simulink model "motor_cc_velocidade_teste"  (R2017b)
settings: Solver=VariableStepAuto  StartTime=0.0  StopTime=10.0  RelTol=1e-3
values from neighbouring files (symbols this model uses):
  b = 0.1    [motor.m]
  J = 0.01    [motor.m]
  Ke = 0.01    [motor.m]
  Kt = 0.01    [motor.m]
  L = 0.5    [motor.m]
  R = 1    [motor.m]
settings Model: Creator=fernandopassold  LastModifiedBy=fernandopassold

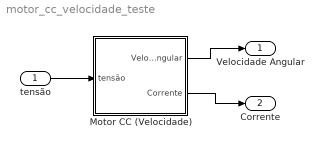
== system motor_cc_velocidade_teste ==
  tensão : Inport
  Motor CC (Velocidade) : Subsystem
  Velocidade Angular : Outport
  Corrente : Outport  Port=2
  wires:
  tensão/1 -> Motor CC (Velocidade)/1(tensão)
  Motor CC (Velocidade)/1(Velocidade Angular) -> Velocidade Angular/1
  Motor CC (Velocidade)/2(Corrente) -> Corrente/1

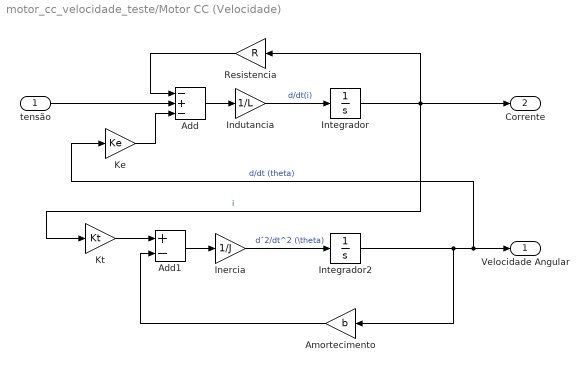
== system motor_cc_velocidade_teste/Motor CC (Velocidade) ==
  tensão : Inport
  Add : Sum  Inputs=-+-
  Add1 : Sum  Inputs=+-
  Amortecimento : Gain  Gain=b
  Indutancia : Gain  Gain=1/L
  Inercia : Gain  Gain=1/J
  Integrador : Integrator
  Integrador2 : Integrator
  Ke : Gain  Gain=Ke
  Kt : Gain  Gain=Kt
  Resistencia : Gain  Gain=R
  Velocidade Angular : Outport
  Corrente : Outport  Port=2
  wires:
  Ke/1 -> Add/3
  Add1/1 -> Inercia/1
  Inercia/1 -> Integrador2/1  "dˆ2/dt^2 (\\theta)"
  Add/1 -> Indutancia/1
  tensão/1 -> Add/2
  Indutancia/1 -> Integrador/1  "d/dt(i)"
  Integrador2/1 -> Velocidade Angular/1, Ke/1, Amortecimento/1  "d/dt (theta)"
  Amortecimento/1 -> Add1/2
  Kt/1 -> Add1/1
  Integrador/1 -> Corrente/1, Kt/1, Resistencia/1  "i"
  Resistencia/1 -> Add/1
